simulink library "SCAN"  (R2016b)
settings: Solver=ode45  StartTime=0.0  StopTime=10.0  RelTol=1e-3  EnableMultiTasking=on
undefined symbols (not defined in the file): CAL_FilterBufferSize, CAL_ROBO_LENG
settings Model: Creator=oelkawok  LastModifiedBy=oelkawok
settings DataIOCC: LimitDataPoints=on
settings OptimizationCC: LifeSpan=inf
settings DebuggingCC: AllowSymbolicDim=off  SFUnexpectedBacktrackingDiag=warning  SFNoUnconditionalDefaultTransitionDiag=warning  SFExecutionAtInitializationDiag=none
settings GRTTargetCC: TargetLangStandard=C89/C90 (ANSI)  GeneratePreprocessorConditionals=Disable all
settings ConfigComp: CovMetricSettings=dw  CovHtmlReporting=on  CovSaveCumulativeToWorkspaceVar=on  CovSaveSingleToWorkspaceVar=on  CovExternalEMLEnable=off

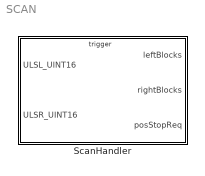
== system SCAN ==
  ScanHandler : Subsystem

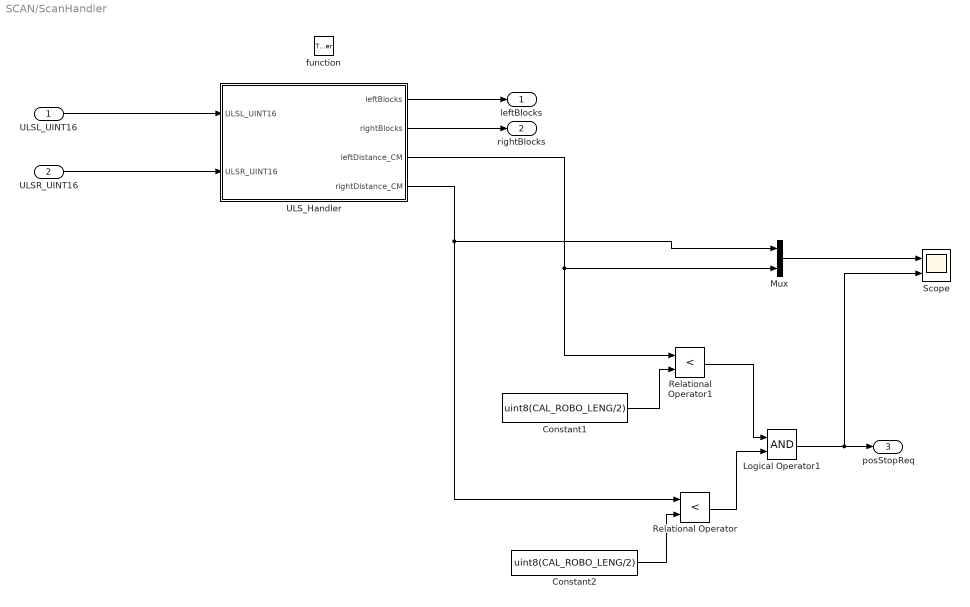
== system SCAN/ScanHandler ==
  ULSL_UINT16 : Inport  PortDimensions=1
  ULSR_UINT16 : Inport  Port=2  PortDimensions=1
  function : TriggerPort  TriggerType=function-call  VariantControl=Variant
  Constant1 : Constant  Value=uint8(CAL_ROBO_LENG/2)
  Constant2 : Constant  Value=uint8(CAL_ROBO_LENG/2)
  Logical Operator1 : Logic  AllPortsSameDT=off  OutDataTypeStr=boolean
  Mux : Mux  Inputs=2
  Relational Operator : RelationalOperator  Operator=<  OutDataTypeStr=boolean  RndMeth=Nearest
  Relational Operator1 : RelationalOperator  Operator=<  OutDataTypeStr=boolean  RndMeth=Nearest
  Scope : Scope  NumInputPorts=2
  ULS_Handler : Subsystem
  leftBlocks : Outport
  rightBlocks : Outport  Port=2
  posStopReq : Outport  Port=3
  wires:
  Mux/1 -> Scope/1
  ULSL_UINT16/1 -> ULS_Handler/1(ULSL_UINT16)
  ULSR_UINT16/1 -> ULS_Handler/2(ULSR_UINT16)
  ULS_Handler/1(leftBlocks) -> leftBlocks/1
  ULS_Handler/2(rightBlocks) -> rightBlocks/1
  Logical Operator1/1 -> posStopReq/1, Scope/2
  Relational Operator/1 -> Logical Operator1/2
  Relational Operator1/1 -> Logical Operator1/1
  ULS_Handler/3(leftDistance_CM) -> Relational Operator1/1, Mux/2
  Constant1/1 -> Relational Operator1/2
  ULS_Handler/4(rightDistance_CM) -> Relational Operator/1, Mux/1
  Constant2/1 -> Relational Operator/2

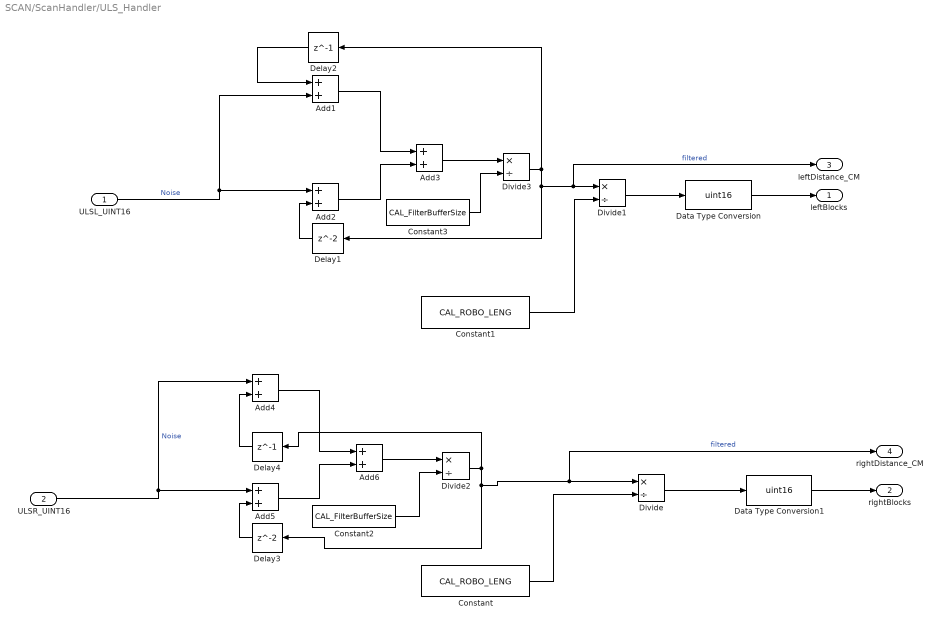
== system SCAN/ScanHandler/ULS_Handler ==
  ULSL_UINT16 : Inport  PortDimensions=1
  ULSR_UINT16 : Inport  Port=2  PortDimensions=1
  Add{1..6} (6 alike) : Sum
  Constant : Constant  Value=CAL_ROBO_LENG
  Constant1 : Constant  Value=CAL_ROBO_LENG
  Constant2 : Constant  Value=CAL_FilterBufferSize  OutDataTypeStr=Inherit: Inherit via back propagation
  Constant3 : Constant  Value=CAL_FilterBufferSize  OutDataTypeStr=Inherit: Inherit via back propagation
  Data Type Conversion : DataTypeConversion  OutDataTypeStr=uint16
  Data Type Conversion1 : DataTypeConversion  OutDataTypeStr=uint16
  Delay1 : Delay  InitialCondition=0
  Delay2 : Delay  DelayLength=1  InitialCondition=0
  Delay3 : Delay  InitialCondition=0
  Delay4 : Delay  DelayLength=1  InitialCondition=0
  Divide : Product  Inputs=*/
  Divide1 : Product  Inputs=*/
  Divide2 : Product  Inputs=*/  OutDataTypeStr=Inherit: Inherit via back propagation
  Divide3 : Product  Inputs=*/  OutDataTypeStr=Inherit: Inherit via back propagation
  leftBlocks : Outport
  rightBlocks : Outport  Port=2
  leftDistance_CM : Outport  Port=3
  rightDistance_CM : Outport  Port=4
  wires:
  Divide2/1 -> Delay4/1, Delay3/1, Divide/1, rightDistance_CM/1  "filtered"
  Constant2/1 -> Divide2/2
  Add6/1 -> Divide2/1
  Add5/1 -> Add6/2
  Add4/1 -> Add6/1
  Delay3/1 -> Add5/2
  ULSR_UINT16/1 -> Add5/1, Add4/1  "Noise"
  Delay4/1 -> Add4/2
  Divide3/1 -> Delay2/1, Delay1/1, Divide1/1, leftDistance_CM/1  "filtered"
  Constant3/1 -> Divide3/2
  Add3/1 -> Divide3/1
  Add2/1 -> Add3/2
  Add1/1 -> Add3/1
  Delay1/1 -> Add2/2
  ULSL_UINT16/1 -> Add2/1, Add1/2  "Noise"
  Delay2/1 -> Add1/1
  Constant/1 -> Divide/2
  Constant1/1 -> Divide1/2
  Divide/1 -> Data Type Conversion1/1
  Divide1/1 -> Data Type Conversion/1
  Data Type Conversion/1 -> leftBlocks/1
  Data Type Conversion1/1 -> rightBlocks/1
